simulink model "Pt_TCon"  (Simulink 7.0)
settings: Solver=ode45  StartTime=0  StopTime=20  FixedStep=TSTEP  RelTol=1e-3
PreLoadFcn:
  | cd extensions\simulink\pt_tcon
  | mengine_carpet_eclass
  | torq_conv_map_eclass
  | Run_ft4wd_eclass
  | cd ..\..\..
undefined symbols (not defined in the file): INV_CAP_TC_TABLE, RM_TC_TABLE
libraries: Solver_SF x1
settings Model: Creator=dhall  LastModifiedBy=ywata  ExtModeTrigMode=oneshot  ExtModeArmWhenConnect=off
settings DataIOCC: LimitDataPoints=off  SaveOutput=off  SaveTime=off  SignalLoggingName=sigsOut
settings OptimizationCC: BooleanDataType=off
settings DebuggingCC: SaveWithParameterizedLinksMsg=none  SignalResolutionControl=TryResolveAllWithWarning  SolverPrmCheckMsg=none  MultiTaskDSMMsg=warning  MultiTaskCondExecSysMsg=none  StrictBusMsg=None
settings HardwareCC: TargetUnknown=on
settings RTWCC: IncludeERTFirstTime=on
settings GRTTargetCC: TargetFcnLib=ansi_tfl_tmw.mat  ModelReferenceCompliant=off  MatFileLogging=off

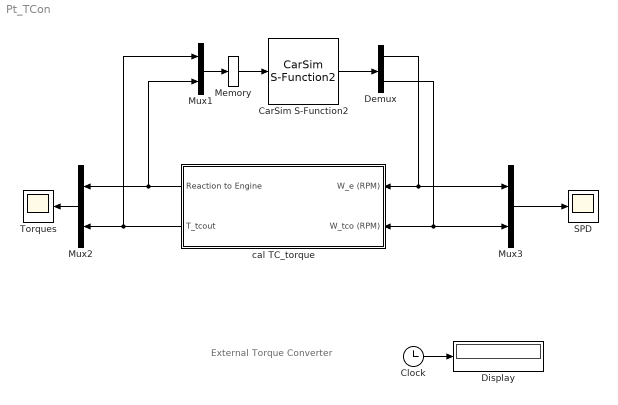
== system Pt_TCon ==
  note: External Torque Converter
  CarSim S-Function2 : Solver_SF/CarSim S-Function2  Priority=1  VehicleCode=???
      settings: AttributesFormatString=Vehicle Code: %<VehicleCode>
  Clock : Clock
      settings: Decimation=10
  Demux : Demux  Outputs=2
  Display : Display
  Memory : Memory
  Mux1 : Mux  Inputs=2
  Mux2 : Mux  Orientation=left  Inputs=2
  Mux3 : Mux  Inputs=2
  SPD : Scope
      settings: TimeRange=20  YMin=0  YMax=6500
  Torques : Scope
      settings: TimeRange=20  YMin=0  YMax=700
  cal TC_torque : Subsystem  Orientation=left
  wires:
  CarSim S-Function2/1 -> Demux/1
  Mux2/1 -> Torques/1
  Mux3/1 -> SPD/1
  Clock/1 -> Display/1
  Mux1/1 -> Memory/1
  Demux/1 -> cal TC_torque/1(W_e (RPM)), Mux3/1
  Demux/2 -> cal TC_torque/2(W_tco (RPM)), Mux3/2
  cal TC_torque/2(T_tcout) -> Mux1/1, Mux2/2
  cal TC_torque/1(Reaction to Engine) -> Mux1/2, Mux2/1
  Memory/1 -> CarSim S-Function2/1

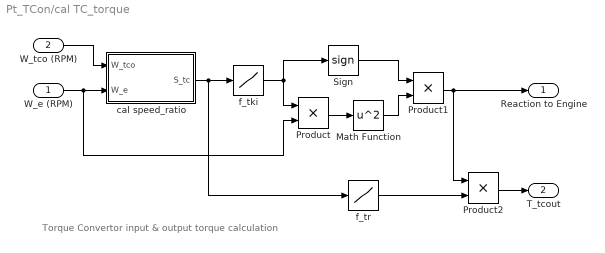
== system Pt_TCon/cal TC_torque ==
  note: Torque Convertor input & output torque calculation
  W_e (RPM) : Inport  OutDataType=sfix(16)  OutScaling=2^0
  W_tco (RPM) : Inport  Port=2  OutDataType=sfix(16)  OutScaling=2^0
  Math Function : Math  Operator=square  SaturateOnIntegerOverflow=on
  Product : Product  OutDataType=sfix(16)  OutScaling=2^0  SaturateOnIntegerOverflow=on  InputSameDT=on
  Product1 : Product  OutDataType=sfix(16)  OutScaling=2^0  SaturateOnIntegerOverflow=on  InputSameDT=on
  Product2 : Product  OutDataType=sfix(16)  OutScaling=2^0  SaturateOnIntegerOverflow=on  InputSameDT=on
  Sign : Signum
  cal speed_ratio : Subsystem
  f_tki : Lookup  InputValues=INV_CAP_TC_TABLE(:,1)  Table=INV_CAP_TC_TABLE(:,2)  OutDataType=sfix(16)  OutScaling=2^0  SaturateOnIntegerOverflow=on
  f_tr : Lookup  InputValues=RM_TC_TABLE(:,1)  Table=RM_TC_TABLE(:,2)  OutDataType=sfix(16)  OutScaling=2^0  SaturateOnIntegerOverflow=on
  Reaction to Engine : Outport
  T_tcout : Outport  Port=2
  wires:
  Product/1 -> Math Function/1
  f_tki/1 -> Product/1, Sign/1
  Math Function/1 -> Product1/2
  Sign/1 -> Product1/1
  W_e (RPM)/1 -> cal speed_ratio/2(W_e), Product/2
  cal speed_ratio/1(S_tc) -> f_tki/1, f_tr/1
  f_tr/1 -> Product2/2
  Product1/1 -> Product2/1, Reaction to Engine/1
  W_tco (RPM)/1 -> cal speed_ratio/1(W_tco)
  Product2/1 -> T_tcout/1

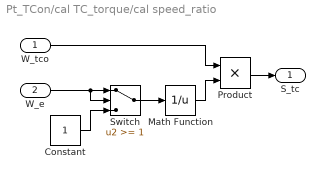
== system Pt_TCon/cal TC_torque/cal speed_ratio ==
  W_tco : Inport  OutDataType=sfix(16)  OutScaling=2^0
  W_e : Inport  Port=2  OutDataType=sfix(16)  OutScaling=2^0
  Constant : Constant  OutDataType=sfix(16)  OutScaling=2^0
  Math Function : Math  Operator=reciprocal  SaturateOnIntegerOverflow=on
  Product : Product  OutDataType=sfix(16)  OutScaling=2^0  SaturateOnIntegerOverflow=on  InputSameDT=on
  Switch : Switch  Threshold=1  SaturateOnIntegerOverflow=on  InputSameDT=on
  S_tc : Outport
  wires:
  Math Function/1 -> Product/2
  W_tco/1 -> Product/1
  Product/1 -> S_tc/1
  Switch/1 -> Math Function/1
  W_e/1 -> Switch/1, Switch/2
  Constant/1 -> Switch/3
